simulink model "lab7_FLC_Pagano"  (R2020a)
settings: Solver=FixedStepAuto  StartTime=0.0  StopTime=400  FixedStep=0.01  RelTol=1e-3
values from neighbouring files (symbols this model uses):
  D = 100    [lab7.mat]
  g = 981    [lab7.mat]
  h_bar = 90    [lab7.mat]
undefined symbols (not defined in the file or in its folder): sigbuilder_block
libraries: simulink x1
settings Model: Creator=bruno  LastModifiedBy=bruno

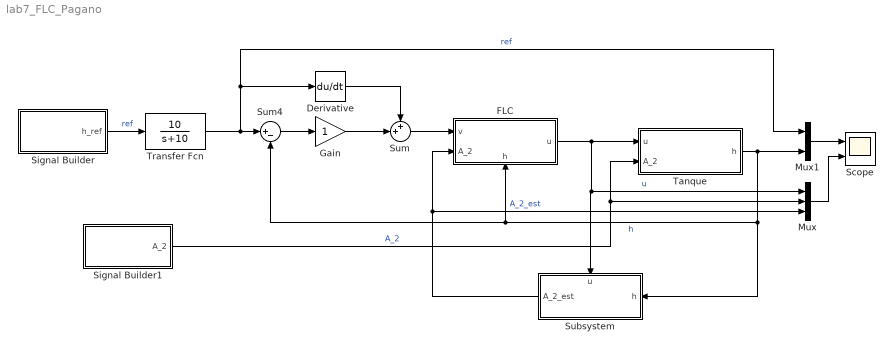
== system lab7_FLC_Pagano ==
  Derivative : Derivative
  FLC : Subsystem
      settings: PortSchema="{\"entries\":[{\"content\":{\"sides\":[{\"content\":{\"connectorIds\":[\"In1\",\"In2\"]},\"type\":\"ConnectorPlacement.EquallySpacedRectSide\",\"uuid\":\"da3e7f5a-9594-4c29-a0ec-3cc1ca63f264\"},{\"content\":{\"connectorIds\":[\"Out1\"],\"side\":\"RIGHT\"},\"type\":\"ConnectorPlacement.EquallySpacedRectSide\",\"uuid\":\"bdfa2608-d653-4e45-a46d-d46342907836\"},{\"content\":{\"connectorIds\":[],\"side\":\"TOP\"},\"type\":\"ConnectorPlacement.EquallySpacedRectSide\",\"uuid\":\"919ad7aa-dcde-46b6-9406-65efd00fdb72\"},{\"content\":{\"connectorIds\":[\"In3\"],\"side\":\"BOTTOM\"},\"type\":\"ConnectorPlacement.EquallySpacedRectSide\",\"uuid\":\"58c39bbf-f8fe-485d-a2fb-a32c56895a64\"}]},\"type\":\"ConnectorPlacement.EquallySpacedConnector\",\"uuid\":\"0132cd69-ef9c-4ff1-92b0-bdee72086be6\"}],\"packageUris\":[\"http://schema.mathworks.com/mf0/Connector/19700101\"],\"version\":\"1.0\"}"
  Gain : Gain
  Mux : Mux  Inputs=3
  Mux1 : Mux  Inputs=2
  Scope : Scope  NumInputPorts=2
  Signal Builder : Subsystem  Tag=STV Subsys  LoadFcn=sigbuilder_block('load');  StartFcn=sigbuilder_block('start');  StopFcn=sigbuilder_block('stop');  ClipboardFcn=sigbuilder_block('clipboard');  mask(Sigbuilder block){tuvar=[0:10]}
      mask help: Simulink:masks:SigbuilderBlock_MD
      mask init:
      | if ~strcmp(get_param(bdroot(gcbh),'SimulationStatus'),'stopped') tuvar = sigbuilder_block('maskInit'); end
      settings: CopyFcn=sigbuilder_block('copy');  DeleteFcn=sigbuilder_block('delete');  ModelCloseFcn=sigbuilder_block('modelClose');  PreSaveFcn=sigbuilder_block('preSave');  PauseFcn=sigbuilder_block('pause');  ContinueFcn=sigbuilder_block('continue');  NameChangeFcn=sigbuilder_block('namechange');  OpenFcn=sigbuilder_block('open',[464.25 220.5 648 331.5 ]);  CloseFcn=sigbuilder_block('close');
      mask Display: plot(0, 0, 100, 100,[2, 2, 32, 32, 2], [68, 8, 8, 68, 68],[32, 2], [38, 38], [32, 19, 2],[53, 60, 44], [32, 17, 17, 2],[16, 16, 31, 31]);txt = getActiveGroup(gcbh);text(2, 100, txt,'verticalAlignment', 'top');
  Signal Builder1 : Subsystem  Tag=STV Subsys  LoadFcn=sigbuilder_block('load');  StartFcn=sigbuilder_block('start');  StopFcn=sigbuilder_block('stop');  ClipboardFcn=sigbuilder_block('clipboard');  mask(Sigbuilder block){tuvar=[0:10]}
      mask help: Simulink:masks:SigbuilderBlock_MD
      mask init:
      | if ~strcmp(get_param(bdroot(gcbh),'SimulationStatus'),'stopped') tuvar = sigbuilder_block('maskInit'); end
      settings: CopyFcn=sigbuilder_block('copy');  DeleteFcn=sigbuilder_block('delete');  ModelCloseFcn=sigbuilder_block('modelClose');  PreSaveFcn=sigbuilder_block('preSave');  PauseFcn=sigbuilder_block('pause');  ContinueFcn=sigbuilder_block('continue');  NameChangeFcn=sigbuilder_block('namechange');  OpenFcn=sigbuilder_block('open',[621.75 239.25 670.5 315.75 ]);  CloseFcn=sigbuilder_block('close');
      mask Display: plot(0, 0, 100, 100,[2, 2, 32, 32, 2], [68, 8, 8, 68, 68],[32, 2], [38, 38], [32, 19, 2],[53, 60, 44], [32, 17, 17, 2],[16, 16, 31, 31]);txt = getActiveGroup(gcbh);text(2, 100, txt,'verticalAlignment', 'top');
  Subsystem : Subsystem
      settings: PortSchema="{\"entries\":[{\"content\":{\"sides\":[{\"content\":{\"connectorIds\":[\"In1\"]},\"type\":\"ConnectorPlacement.EquallySpacedRectSide\",\"uuid\":\"f3ee839e-5dfb-44a5-9b76-652e849a55f5\"},{\"content\":{\"connectorIds\":[\"Out1\"],\"side\":\"RIGHT\"},\"type\":\"ConnectorPlacement.EquallySpacedRectSide\",\"uuid\":\"bbe81370-0c45-427a-bd58-27f952b30e92\"},{\"content\":{\"connectorIds\":[\"In2\"],\"side\":\"TOP\"},\"type\":\"ConnectorPlacement.EquallySpacedRectSide\",\"uuid\":\"f6dcd5ca-c5f4-4a96-9ca1-58a39393d7a4\"}]},\"type\":\"ConnectorPlacement.EquallySpacedConnector\",\"uuid\":\"1ad53398-b949-437a-aa87-04b8756a46bc\"}],\"packageUris\":[\"http://schema.mathworks.com/mf0/Connector/19700101\"],\"version\":\"1.0\"}"
  Sum : Sum  Inputs=++|
  Sum4 : Sum  Inputs=|+-
  Tanque : Subsystem
  Transfer Fcn : TransferFcn  Numerator=[10]  Denominator=[1 10]
  wires:
  Tanque/1(h) -> Mux1/2, Subsystem/1(h), Sum4/2, FLC/3(h)  "h"
  Transfer Fcn/1 -> Mux1/1, Derivative/1, Sum4/1  "ref"
  Mux1/1 -> Scope/1
  Signal Builder1/1(A_2) -> Mux/2, Tanque/2(A_2)  "A_2"
  FLC/1(u) -> Subsystem/2(u), Mux/1, Tanque/1(u)  "u"
  Signal Builder/1(h_ref) -> Transfer Fcn/1  "ref"
  Derivative/1 -> Sum/1
  Sum/1 -> FLC/1(v)
  Sum4/1 -> Gain/1
  Gain/1 -> Sum/2
  Subsystem/1(A_2_est) -> Mux/3, FLC/2(A_2)  "A_2_est"
  Mux/1 -> Scope/2

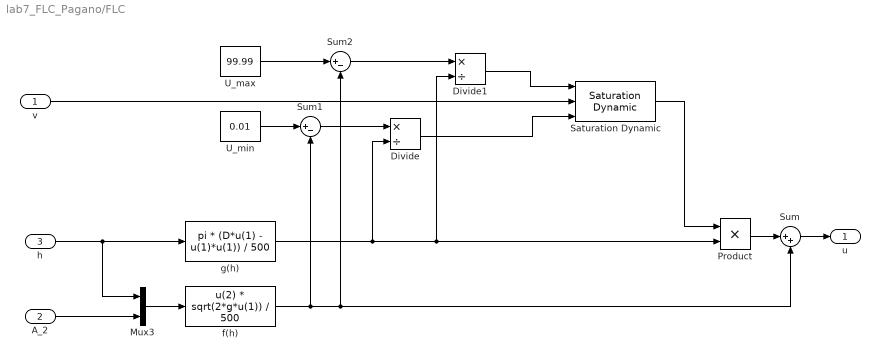
== system lab7_FLC_Pagano/FLC ==
  v : Inport
  A_2 : Inport  Port=2
  h : Inport  Port=3
  Divide : Product  Inputs=*/
  Divide1 : Product  Inputs=*/
  Mux3 : Mux  Inputs=2
  Product : Product
  Saturation Dynamic : simulink/Discontinuities/Saturation Dynamic  OutMin=[]  OutMax=[]  OutDataTypeStr=Inherit: Same as second input  OutDataType=fixdt(1, 16)  OutScaling=2^-10  DoSatur=off
  Sum : Sum  Inputs=|++
  Sum1 : Sum  Inputs=|+-
  Sum2 : Sum  Inputs=|+-
  U_max : Constant  Value=99.99
  U_min : Constant  Value=0.01
  f(h) : Fcn  Expr=u(2) * sqrt(2*g*u(1)) / 500
  g(h) : Fcn  Expr=pi * (D*u(1) - u(1)*u(1)) / 500
  u : Outport
  wires:
  h/1 -> g(h)/1, Mux3/1
  Mux3/1 -> f(h)/1
  A_2/1 -> Mux3/2
  g(h)/1 -> Divide/2, Divide1/2, Product/2
  Sum/1 -> u/1
  Product/1 -> Sum/1
  f(h)/1 -> Sum1/2, Sum/2, Sum2/2
  v/1 -> Saturation Dynamic/2
  U_min/1 -> Sum1/1
  U_max/1 -> Sum2/1
  Saturation Dynamic/1 -> Product/1
  Sum1/1 -> Divide/1
  Divide/1 -> Saturation Dynamic/3
  Sum2/1 -> Divide1/1
  Divide1/1 -> Saturation Dynamic/1

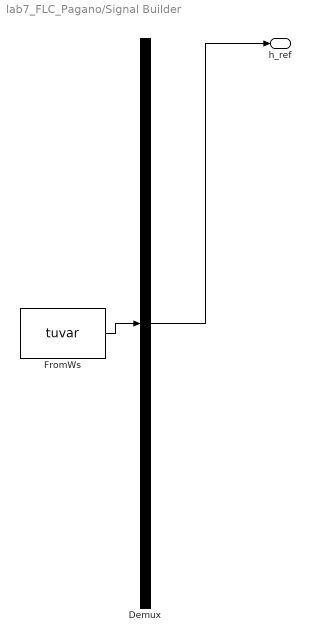
== system lab7_FLC_Pagano/Signal Builder ==
  Demux : Demux  Tag=STV Demux  Outputs=1
      settings: DisplayOption=none
  FromWs : FromWorkspace  Tag=STV FromWs  VariableName=tuvar
      SigBuilderData=|
      | common.afterFinalStr = 'Extrapolate'
      | common.sampleTime = 0
      | dataSet.timeRange = [0 400]
      | dataSet.name = 'Group 1'
      | sbobj.Groups.Name = 'Group 1'
      | sbobj.Groups.Signals.Name = 'h_ref'
      | sbobj.Groups.Signals.XData = [0 50 50 150 150 250 250 300 300 400]
      | sbobj.Groups.Signals.YData = [90 90 50 50 10 10 50 50 90 90]
      | sbobj.Groups.TimeRange = [0 400]
  h_ref : Outport  Tag=STV Outport
  wires:
  Demux/1 -> h_ref/1
  FromWs/1 -> Demux/1

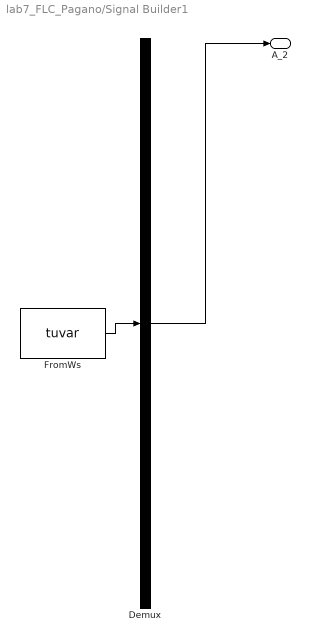
== system lab7_FLC_Pagano/Signal Builder1 ==
  Demux : Demux  Tag=STV Demux  Outputs=1
      settings: DisplayOption=none
  FromWs : FromWorkspace  Tag=STV FromWs  VariableName=tuvar
      SigBuilderData=|
      | common.afterFinalStr = 'Extrapolate'
      | common.sampleTime = 0
      | dataSet.timeRange = [0 400]
      | dataSet.name = 'Group 1'
      | sbobj.Groups.Name = 'Group 1'
      | sbobj.Groups.Signals.Name = 'A_2'
      | sbobj.Groups.Signals.XData = [0 100 100 150 150 350 350 375 400]
      | sbobj.Groups.Signals.YData = [19.6 19.6 9.8 9.8 19.6 19.6 10 10 10]
      | sbobj.Groups.TimeRange = [0 400]
  A_2 : Outport  Tag=STV Outport
  wires:
  Demux/1 -> A_2/1
  FromWs/1 -> Demux/1

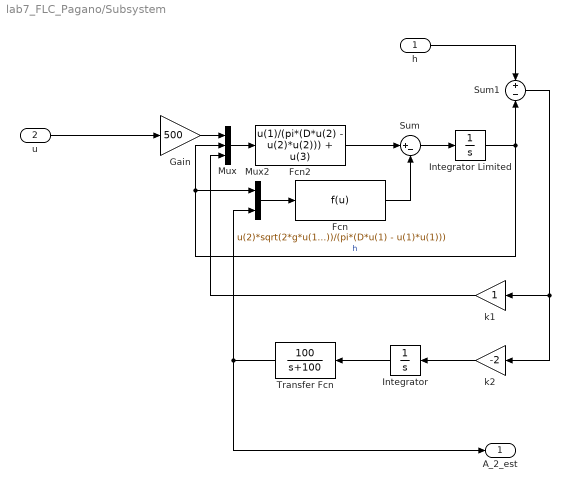
== system lab7_FLC_Pagano/Subsystem ==
  h : Inport
  u : Inport  Port=2
  Fcn : Fcn  Expr=u(2)*sqrt(2*g*u(1))/(pi*(D*u(1) - u(1)*u(1)))
  Fcn2 : Fcn  Expr=u(1)/(pi*(D*u(2) - u(2)*u(2))) + u(3)
  Gain : Gain  Gain=500
  Integrator : Integrator
  Integrator Limited : Integrator  InitialCondition=h_bar  LimitOutput=on  UpperSaturationLimit=100-0.001  LowerSaturationLimit=0.001
  Mux : Mux  Inputs=3
  Mux2 : Mux  Inputs=2
  Sum : Sum  Inputs=|+-
  Sum1 : Sum  Inputs=+|-
  Transfer Fcn : TransferFcn  Numerator=[100]  Denominator=[1 100]
  k1 : Gain
  k2 : Gain  Gain=-2
  A_2_est : Outport
  wires:
  Fcn/1 -> Sum/2
  Transfer Fcn/1 -> Mux2/2, A_2_est/1
  Sum/1 -> Integrator Limited/1
  Fcn2/1 -> Sum/1
  Integrator Limited/1 -> Mux2/1, Mux/2, Sum1/2  "h"
  Mux2/1 -> Fcn/1
  Mux/1 -> Fcn2/1
  Gain/1 -> Mux/1
  u/1 -> Gain/1
  h/1 -> Sum1/1
  Sum1/1 -> k2/1, k1/1
  k1/1 -> Mux/3
  k2/1 -> Integrator/1
  Integrator/1 -> Transfer Fcn/1

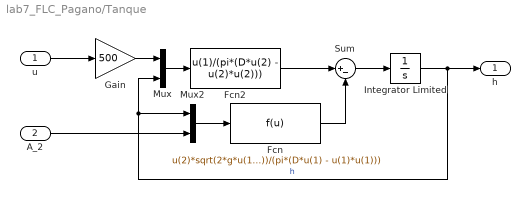
== system lab7_FLC_Pagano/Tanque ==
  u : Inport
  A_2 : Inport  Port=2
  Fcn : Fcn  Expr=u(2)*sqrt(2*g*u(1))/(pi*(D*u(1) - u(1)*u(1)))
  Fcn2 : Fcn  Expr=u(1)/(pi*(D*u(2) - u(2)*u(2)))
  Gain : Gain  Gain=500
  Integrator Limited : Integrator  InitialCondition=h_bar  LimitOutput=on  UpperSaturationLimit=100-0.001  LowerSaturationLimit=0.001
  Mux : Mux  Inputs=2
  Mux2 : Mux  Inputs=2
  Sum : Sum  Inputs=|+-
  h : Outport
  wires:
  Integrator Limited/1 -> h/1, Mux2/1, Mux/2  "h"
  Sum/1 -> Integrator Limited/1
  Mux/1 -> Fcn2/1
  A_2/1 -> Mux2/2
  Mux2/1 -> Fcn/1
  Fcn/1 -> Sum/2
  Fcn2/1 -> Sum/1
  Gain/1 -> Mux/1
  u/1 -> Gain/1
